simulink library "tethersMoment_cl"  (R2018b)
settings: Solver=VariableStepAuto  StartTime=0.0  StopTime=10.0  RelTol=1e-3
undefined symbols (not defined in the file or in its folder): arms
libraries: vrlib x1
settings Model: Creator=mcobb  LastModifiedBy=mcobb

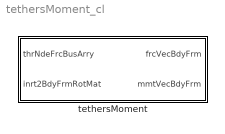
== system tethersMoment_cl ==
  tethersMoment : Subsystem  mask{arms=arms}
      mask prompts: arms "Moment arm(s)"

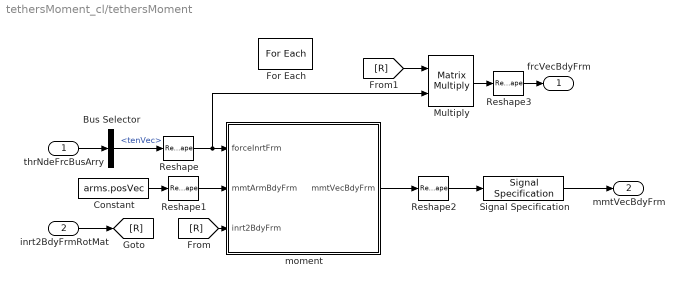
== system tethersMoment_cl/tethersMoment ==
  thrNdeFrcBusArry : Inport  Partition=on  PartitionDimension=1  PartitionWidth=1  PartitionOffset=0
  inrt2BdyFrmRotMat : Inport  Port=2
  Bus Selector : BusSelector  OutputSignals=tenVec
  Constant : Constant  Value=arms.posVec
  For Each : ForEach  DisableCoverage=on  IterateSubsysMaskParameter=on  SubsysMaskParameterIterationDimension=2  IndexMode=One-based
  Multiply : Product  Multiplication=Matrix(*)
  Reshape{,1..3} (4 alike) : Reshape  OutputDimensionality=Column vector (2-D)
  Signal Specification : SignalSpecification  Dimensions=[3 1]
  moment : Subsystem
  frcVecBdyFrm : Outport  ConcatenationDimension=2
  mmtVecBdyFrm : Outport  Port=2  ConcatenationDimension=2
  wires:
  moment/1(mmtVecBdyFrm) -> Reshape2/1
  thrNdeFrcBusArry/1 -> Bus Selector/1
  inrt2BdyFrmRotMat/1 -> [R]
  Constant/1 -> Reshape1/1
  Bus Selector/1 -> Reshape/1  "<tenVec>"
  [R] -> moment/3(inrt2BdyFrm)
  Multiply/1 -> Reshape3/1
  [R] -> Multiply/1
  Reshape/1 -> Multiply/2, moment/1(forceInrtFrm)
  Reshape1/1 -> moment/2(mmtArmBdyFrm)
  Reshape2/1 -> Signal Specification/1
  Reshape3/1 -> frcVecBdyFrm/1
  Signal Specification/1 -> mmtVecBdyFrm/1

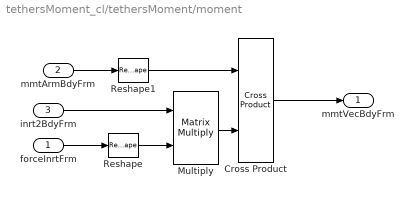
== system tethersMoment_cl/tethersMoment/moment ==
  forceInrtFrm : Inport
  mmtArmBdyFrm : Inport  Port=2
  inrt2BdyFrm : Inport  Port=3
  Cross Product : vrlib/Utilities/Cross Product
      settings: SourceProductBaseCode=VR
  Multiply : Product  Multiplication=Matrix(*)
  Reshape : Reshape  OutputDimensionality=Column vector (2-D)
  Reshape1 : Reshape  OutputDimensionality=Column vector (2-D)
  mmtVecBdyFrm : Outport
  wires:
  Reshape1/1 -> Cross Product/1
  Reshape/1 -> Multiply/2
  Cross Product/1 -> mmtVecBdyFrm/1
  mmtArmBdyFrm/1 -> Reshape1/1
  Multiply/1 -> Cross Product/2
  inrt2BdyFrm/1 -> Multiply/1
  forceInrtFrm/1 -> Reshape/1
